simulink model "p_packetizer_test"  (R2012b)
settings: Solver=ode45  StartTime=0.0  StopTime=16384 * 8  RelTol=1e-3
libraries: xbsIndex_r4 x583, casper_library_misc x4
(part 1 of 4)
settings Model: Creator=jackh  LastModifiedBy=jackh

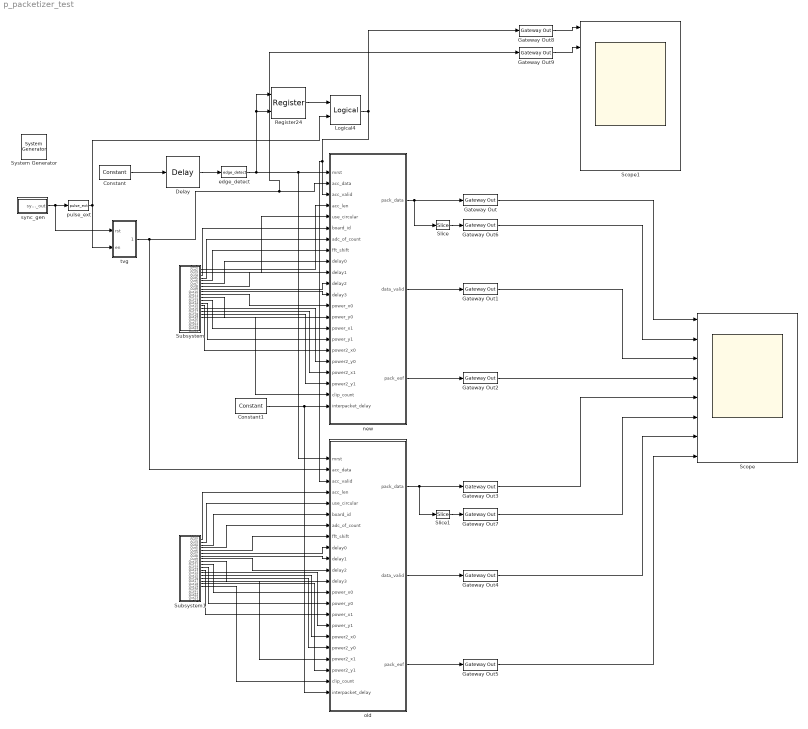
== system p_packetizer_test ==
  " System Generator" : xbsIndex_r4/ System Generator  Tag=genX  xilinxfamily=virtex6  part=xc6vsx475t  speed=-1  package=ff1759  synthesis_tool=XST  clock_wrapper=Clock Enables  directory=./eovsa_corr/sysgen  proj_type=Project Navigator  Synth_file=XST Defaults  Impl_file=ISE Defaults  testbench=off  simulink_period=1  sysclk_period=5  dcm_input_clock_period=100  incr_netlist=off  trim_vbits=Everywhere in SubSystem  dbl_ovrd=According to Block Masks  core_generation=According to Block Masks  run_coregen=off  deprecated_control=off  eval_field=0  block_type=sysgen
      settings: block_version=11.4
  Constant : xbsIndex_r4/Constant  const=1  gui_display_data_type=Boolean  arith_type=Boolean  n_bits=16  bin_pt=14  preci_type=Single  exp_width=8  frac_width=24  explicit_period=on  period=1  equ=P=C  opselect=C  inp2=PCIN>>17  opr=+  inp1=P  carry=CIN  dbl_ovrd=off  block_type=constant
  Constant1 : xbsIndex_r4/Constant  const=5  gui_display_data_type=Fixed-point  arith_type=Unsigned  n_bits=16  bin_pt=0  preci_type=Single  exp_width=8  frac_width=24  explicit_period=on  period=1  equ=P=C  opselect=C  inp2=PCIN>>17  opr=+  inp1=P  carry=CIN  dbl_ovrd=off  block_type=constant
  Delay : xbsIndex_r4/Delay  rst=off  infoeditControl=Selection of Reset will increase slice count due to use of real FFs and instead of SRLs  en=off  latency=3000  dbl_ovrd=off  reg_retiming=off  block_type=delay
  Gateway Out{,1..9} (10 alike) : xbsIndex_r4/Gateway Out  inherit_from_input=off  hdl_port=on  timing_constraint=None  locs_specified=off  LOCs={}  UseAsDAC=off  DACChannel='1'  block_type=gatewayout
  Logical4 : xbsIndex_r4/Logical  logical_function=AND  inputs=2  en=off  latency=0  precision=Full  arith_type=Unsigned  n_bits=16  bin_pt=0  align_bp=on  dbl_ovrd=off  block_type=logical
      settings: block_version=11.4
  Register24 : xbsIndex_r4/Register  init=0  rst=off  en=on  dbl_ovrd=off  block_type=register
  Scope : Scope  NumInputPorts=8
      settings: YMin=0~0~0~0~0~0~0~0  YMax=7e+18~4500~1~1~7e+18~4500~1~1
  Scope1 : Scope  NumInputPorts=8
      settings: YMin=0~0~0~0~0~0~0~0  YMax=7e+18~4500~1~1~7e+18~4500~1~1  SaveName=ScopeData2
  Slice : xbsIndex_r4/Slice  nbits=13  boolean_output=off  mode=Lower Bit Location + Width  bit1=0  base1=MSB of Input  bit0=0  base0=LSB of Input  dbl_ovrd=off  block_type=slice
  Slice1 : xbsIndex_r4/Slice  nbits=13  boolean_output=off  mode=Lower Bit Location + Width  bit1=0  base1=MSB of Input  bit0=0  base0=LSB of Input  dbl_ovrd=off  block_type=slice
  Subsystem : Subsystem
  Subsystem1 : Subsystem
  edge_detect : casper_library_misc/edge_detect  edge=Rising  polarity=Active High  x_in=[0 0.08 0.08 0.16 0.16 0.24 0.24 0.32 0.32 0.4]  y_in="[-1 -1  1  1  1  1  1  1  1  1]"  x_out=[0.6 0.68 0.68 0.76 0.76 0.84 0.84 0.92 0.92 1]  y_out="[-1 -1  1  1 -1 -1 -1 -1 -1 -1]"
  new : Subsystem  mask{header_len=88, n_packets=256, freq_chan=12}
      mask prompts: header_len "Packet header length (bytes)"; n_packets "No. of packets per accumulation"; freq_chan "Total frequency channels ( 2 ^ ? )"
      mask init:
      | data_len = (2 ^ freq_chan) * 4 * (96 / 8 ) / n_packets;
  old : Subsystem  mask{header_len=88, n_packets=256, freq_chan=12}
      mask prompts: header_len "Packet header length (bytes)"; n_packets "No. of packets per accumulation"; freq_chan "Total frequency channels ( 2 ^ ? )"
      mask init:
      | data_len = (2 ^ freq_chan) * 4 * (96 / 8 ) / n_packets;
  pulse_ext : casper_library_misc/pulse_ext  pulse_len=2048
  sync_gen : Subsystem  AncestorBlock=casper_library_misc/sync_gen  mask(sync_gen){sim_acc_len=16, fft_size=2048, fft_simult_inputs=1, pfb_fir_taps=1, reorder_vec=[1], scale=1}
      mask prompts: sim_acc_len "Simulation Accumulation Length"; fft_size "FFT Size"; fft_simult_inputs "Simultaneous Inputs (FFT)"; pfb_fir_taps "Taps in pfb_fir (use 1 if no pfb_fir)"; reorder_vec "Reorder Orders (e.g. [2 2 2])"
      mask help:
      | This block computes the sync period based on system parameters as
      | described in Casper memo.  Detailed descritions of the block's
      | variables can be found in the 'Block Documentation' section of
      | the CASPER wiki.
      mask init:
      | sync_gen_init(gcb, ...
      |     'sim_acc_len', sim_acc_len, ...
      |     'fft_size', fft_size, ...
      |     'fft_simult_inputs', fft_simult_inputs,...
      |     'pfb_fir_taps', pfb_fir_taps, ...
      |     'reorder_vec', reorder_vec, ...
      |     'scale', scale);
      settings: AttributesFormatString=sim_sync_period=32768
      mask Help:
      | SyncPeriod=LCM(reorder_vec)*(acc_num)*(pfb_fir_len)*(fft_size/fft_simult_inputs)
      | 
      | See CASPER sync pulse memo for more details.
  tvg : Subsystem
  wires:
  Constant/1 -> Delay/1
  Delay/1 -> edge_detect/1
  edge_detect/1 -> Register24/2, Register24/1, old/1(mrst), new/1(mrst)
  sync_gen/1(sync_out) -> tvg/1(rst), pulse_ext/1
  pulse_ext/1 -> tvg/2(en), Logical4/2
  Constant1/1 -> old/22(interpacket_delay), new/22(interpacket_delay)
  Subsystem/10(Out10) -> new/12(delay3)
  Subsystem/9(Out9) -> new/11(delay2)
  Subsystem/11(Out11) -> new/13(power_x0)
  Subsystem/8(Out8) -> new/10(delay1)
  Subsystem/12(Out12) -> new/14(power_y0)
  Subsystem/7(Out7) -> new/9(delay0)
  Subsystem/13(Out13) -> new/15(power_x1)
  Subsystem/6(Out6) -> new/8(fft_shift)
  Subsystem/14(Out14) -> new/16(power_y1)
  Subsystem/5(Out5) -> new/7(adc_of_count)
  Subsystem/15(Out15) -> new/17(power2_x0)
  Subsystem/4(Out4) -> new/6(board_id)
  Subsystem/16(Out16) -> new/18(power2_y0)
  Subsystem/3(Out3) -> new/5(use_circular)
  Subsystem/17(Out17) -> new/19(power2_x1)
  Subsystem/2(Out2) -> new/4(acc_len)
  Subsystem/18(Out18) -> new/20(power2_y1)
  Subsystem/19(Out19) -> new/21(clip_count)
  Subsystem1/8(Out8) -> old/10(delay1)
  Subsystem1/7(Out7) -> old/9(delay0)
  Subsystem1/9(Out9) -> old/11(delay2)
  Subsystem1/6(Out6) -> old/8(fft_shift)
  Subsystem1/10(Out10) -> old/12(delay3)
  Subsystem1/5(Out5) -> old/7(adc_of_count)
  Subsystem1/11(Out11) -> old/13(power_x0)
  Subsystem1/4(Out4) -> old/6(board_id)
  Subsystem1/12(Out12) -> old/14(power_y0)
  Subsystem1/3(Out3) -> old/5(use_circular)
  Subsystem1/13(Out13) -> old/15(power_x1)
  Subsystem1/2(Out2) -> old/4(acc_len)
  Subsystem1/14(Out14) -> old/16(power_y1)
  Subsystem1/15(Out15) -> old/17(power2_x0)
  Subsystem1/16(Out16) -> old/18(power2_y0)
  Subsystem1/17(Out17) -> old/19(power2_x1)
  Subsystem1/18(Out18) -> old/20(power2_y1)
  Subsystem1/19(Out19) -> old/21(clip_count)
  new/1(pack_data) -> Slice/1, Gateway Out/1
  new/2(data_valid) -> Gateway Out1/1
  new/3(pack_eof) -> Gateway Out2/1
  old/1(pack_data) -> Slice1/1, Gateway Out3/1
  old/2(data_valid) -> Gateway Out4/1
  old/3(pack_eof) -> Gateway Out5/1
  tvg/1(Out1) -> old/2(acc_data), Gateway Out9/1, new/2(acc_data)
  Slice/1 -> Gateway Out6/1
  Slice1/1 -> Gateway Out7/1
  Gateway Out3/1 -> Scope/5
  Gateway Out7/1 -> Scope/6
  Gateway Out2/1 -> Scope/4
  Gateway Out4/1 -> Scope/7
  Gateway Out1/1 -> Scope/3
  Gateway Out5/1 -> Scope/8
  Gateway Out6/1 -> Scope/2
  Gateway Out/1 -> Scope/1
  Register24/1 -> Logical4/1
  Logical4/1 -> old/3(acc_valid), new/3(acc_valid), Gateway Out8/1
  Gateway Out8/1 -> Scope1/1
  Gateway Out9/1 -> Scope1/2

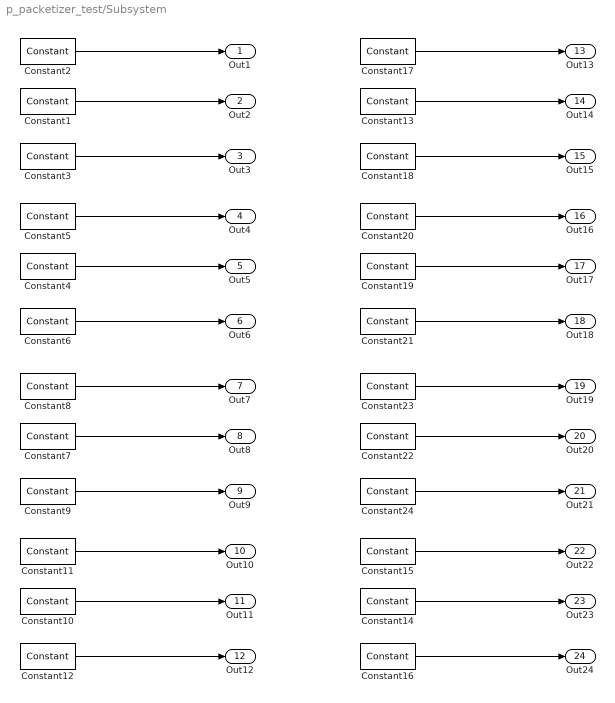
== system p_packetizer_test/Subsystem ==
  Constant{1..24} (24 alike) : xbsIndex_r4/Constant  const=1  gui_display_data_type=Fixed-point  arith_type=Unsigned  n_bits=32  bin_pt=0  preci_type=Single  exp_width=8  frac_width=24  explicit_period=on  period=1  equ=P=C  opselect=C  inp2=PCIN>>17  opr=+  inp1=P  carry=CIN  dbl_ovrd=off  block_type=constant
  Out1 : Outport
  Out2 : Outport  Port=2
  Out3 : Outport  Port=3
  Out4 : Outport  Port=4
  Out5 : Outport  Port=5
  Out6 : Outport  Port=6
  Out7 : Outport  Port=7
  Out8 : Outport  Port=8
  Out9 : Outport  Port=9
  Out10 : Outport  Port=10
  Out11 : Outport  Port=11
  Out12 : Outport  Port=12
  Out13 : Outport  Port=13
  Out14 : Outport  Port=14
  Out15 : Outport  Port=15
  Out16 : Outport  Port=16
  Out17 : Outport  Port=17
  Out18 : Outport  Port=18
  Out19 : Outport  Port=19
  Out20 : Outport  Port=20
  Out21 : Outport  Port=21
  Out22 : Outport  Port=22
  Out23 : Outport  Port=23
  Out24 : Outport  Port=24
  wires:
  Constant2/1 -> Out1/1
  Constant1/1 -> Out2/1
  Constant3/1 -> Out3/1
  Constant5/1 -> Out4/1
  Constant4/1 -> Out5/1
  Constant6/1 -> Out6/1
  Constant8/1 -> Out7/1
  Constant7/1 -> Out8/1
  Constant9/1 -> Out9/1
  Constant11/1 -> Out10/1
  Constant10/1 -> Out11/1
  Constant12/1 -> Out12/1
  Constant17/1 -> Out13/1
  Constant13/1 -> Out14/1
  Constant18/1 -> Out15/1
  Constant20/1 -> Out16/1
  Constant19/1 -> Out17/1
  Constant21/1 -> Out18/1
  Constant23/1 -> Out19/1
  Constant22/1 -> Out20/1
  Constant24/1 -> Out21/1
  Constant15/1 -> Out22/1
  Constant14/1 -> Out23/1
  Constant16/1 -> Out24/1

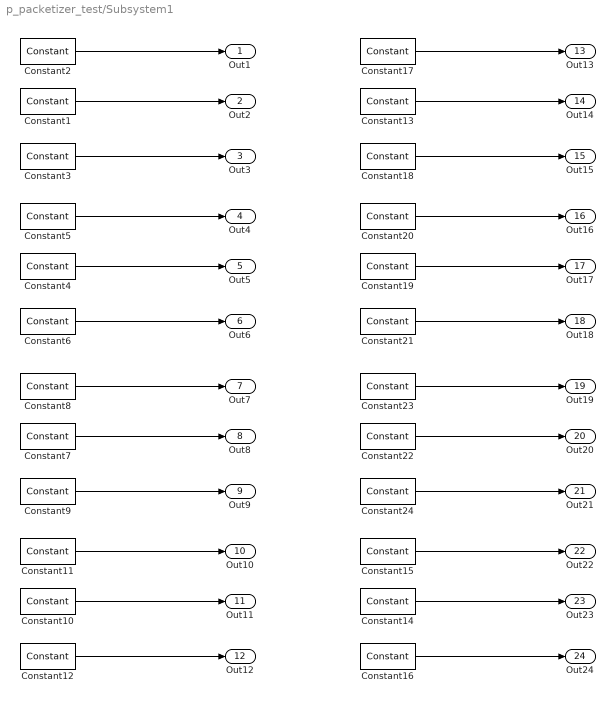
== system p_packetizer_test/Subsystem1 ==
  Constant{1..24} (24 alike) : xbsIndex_r4/Constant  const=1  gui_display_data_type=Fixed-point  arith_type=Unsigned  n_bits=32  bin_pt=0  preci_type=Single  exp_width=8  frac_width=24  explicit_period=on  period=1  equ=P=C  opselect=C  inp2=PCIN>>17  opr=+  inp1=P  carry=CIN  dbl_ovrd=off  block_type=constant
  Out1 : Outport
  Out2 : Outport  Port=2
  Out3 : Outport  Port=3
  Out4 : Outport  Port=4
  Out5 : Outport  Port=5
  Out6 : Outport  Port=6
  Out7 : Outport  Port=7
  Out8 : Outport  Port=8
  Out9 : Outport  Port=9
  Out10 : Outport  Port=10
  Out11 : Outport  Port=11
  Out12 : Outport  Port=12
  Out13 : Outport  Port=13
  Out14 : Outport  Port=14
  Out15 : Outport  Port=15
  Out16 : Outport  Port=16
  Out17 : Outport  Port=17
  Out18 : Outport  Port=18
  Out19 : Outport  Port=19
  Out20 : Outport  Port=20
  Out21 : Outport  Port=21
  Out22 : Outport  Port=22
  Out23 : Outport  Port=23
  Out24 : Outport  Port=24
  wires:
  Constant16/1 -> Out24/1
  Constant14/1 -> Out23/1
  Constant15/1 -> Out22/1
  Constant24/1 -> Out21/1
  Constant22/1 -> Out20/1
  Constant23/1 -> Out19/1
  Constant21/1 -> Out18/1
  Constant19/1 -> Out17/1
  Constant20/1 -> Out16/1
  Constant18/1 -> Out15/1
  Constant13/1 -> Out14/1
  Constant17/1 -> Out13/1
  Constant12/1 -> Out12/1
  Constant10/1 -> Out11/1
  Constant11/1 -> Out10/1
  Constant9/1 -> Out9/1
  Constant7/1 -> Out8/1
  Constant8/1 -> Out7/1
  Constant6/1 -> Out6/1
  Constant4/1 -> Out5/1
  Constant5/1 -> Out4/1
  Constant3/1 -> Out3/1
  Constant1/1 -> Out2/1
  Constant2/1 -> Out1/1

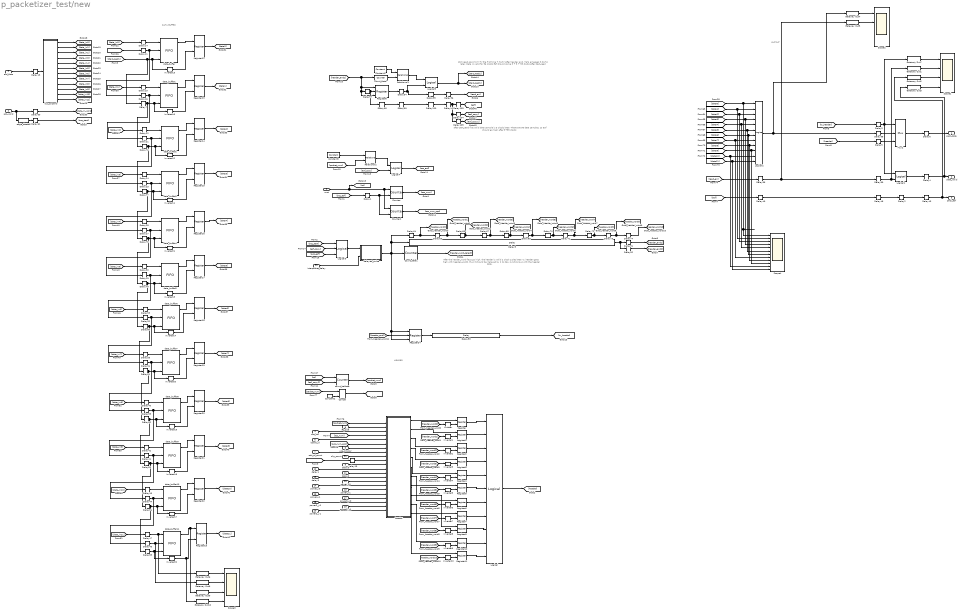
== system p_packetizer_test/new ==
  note: After the header_word flags go high, the header is valid 2 clock cycles later.
      | tx_header goes high with header_word0, thus it should be delayed by 2 to stay synchronous with the header data.
  note: after start_read first valid data sample is 3 clocks later.
      | There are 96 data samples, so eof should go high after 3+95 clocks
  note: start_read goes high for the first time 3 clocks after header_end.
      | Data emerges 3 clocks later.
      | Data is valid for 96 clocks
      | Eof should come 3 + 3 + 95 clocks after start_read
  note: OUTPUT
  note: HEADER
  note: DATA BUFFER
  mrst : Inport
  acc_data : Inport  Port=2
  acc_valid : Inport  Port=3
  acc_len : Inport  Port=4
  use_circular : Inport  Port=5
  board_id : Inport  Port=6
  adc_of_count : Inport  Port=7
  fft_shift : Inport  Port=8
  delay0 : Inport  Port=9
  delay1 : Inport  Port=10
  delay2 : Inport  Port=11
  delay3 : Inport  Port=12
  power_x0 : Inport  Port=13
  power_y0 : Inport  Port=14
  power_x1 : Inport  Port=15
  power_y1 : Inport  Port=16
  power2_x0 : Inport  Port=17
  power2_y0 : Inport  Port=18
  power2_x1 : Inport  Port=19
  power2_y1 : Inport  Port=20
  clip_count : Inport  Port=21
  interpacket_delay : Inport  Port=22
  Concat : xbsIndex_r4/Concat  num_inputs=2  dbl_ovrd=off  block_type=concat
  Constant1 : xbsIndex_r4/Constant  const=0  gui_display_data_type=Fixed-point  arith_type=Unsigned  n_bits=4  bin_pt=0  preci_type=Single  exp_width=8  frac_width=24  explicit_period=on  period=1  equ=P=C  opselect=C  inp2=PCIN>>17  opr=+  inp1=P  carry=CIN  dbl_ovrd=off  block_type=constant
      settings: block_version=11.4
  Constant2 : xbsIndex_r4/Constant  const=0  gui_display_data_type=Fixed-point  arith_type=Unsigned  n_bits=log2( (2 ^ freq_chan) / n_packets )  bin_pt=0  preci_type=Single  exp_width=8  frac_width=24  explicit_period=on  period=1  equ=P=C  opselect=C  inp2=PCIN>>17  opr=+  inp1=P  carry=CIN  dbl_ovrd=off  block_type=constant
      settings: block_version=11.4
  Constant3 : xbsIndex_r4/Constant  const=n_packets - 1  gui_display_data_type=Fixed-point  arith_type=Unsigned  n_bits=ceil( log2( n_packets - 1 ) )  bin_pt=0  preci_type=Single  exp_width=8  frac_width=24  explicit_period=on  period=1  equ=P=C  opselect=C  inp2=PCIN>>17  opr=+  inp1=P  carry=CIN  dbl_ovrd=off  block_type=constant
      settings: block_version=11.4
  Count_data1 : xbsIndex_r4/Counter  cnt_type=Count Limited  cnt_to=header_len / 8 - 1  operation=Up  start_count=0  cnt_by_val=1  arith_type=Unsigned  n_bits=ceil( log2( header_len / 8 - 1 ) )  bin_pt=0  load_pin=off  rst=on  en=off  explicit_period=on  period=1  dbl_ovrd=off  use_behavioral_HDL=on  implementation=Fabric  use_rpm=off  block_type=counter
  Count_data7 : xbsIndex_r4/Counter  cnt_type=Count Limited  cnt_to=11  operation=Up  start_count=0  cnt_by_val=1  arith_type=Unsigned  n_bits=4  bin_pt=0  load_pin=off  rst=on  en=off  explicit_period=on  period=1  dbl_ovrd=off  use_behavioral_HDL=on  implementation=Fabric  use_rpm=off  block_type=counter
  Counter : xbsIndex_r4/Counter  cnt_type=Free Running  cnt_to=Inf  operation=Up  start_count=0  cnt_by_val=1  arith_type=Unsigned  n_bits=32  bin_pt=0  load_pin=off  rst=on  en=on  explicit_period=off  period=1  dbl_ovrd=off  use_behavioral_HDL=off  implementation=DSP48  block_type=counter
      settings: block_version=11.4
  Counter1 : xbsIndex_r4/Counter  cnt_type=Count Limited  cnt_to=49  operation=Up  start_count=0  cnt_by_val=1  arith_type=Unsigned  n_bits=8  bin_pt=0  load_pin=off  rst=on  en=on  explicit_period=off  period=1  dbl_ovrd=off  use_behavioral_HDL=off  implementation=Fabric  block_type=counter
      settings: block_version=11.4
  Delay{1..4,6,9,13..14,32,34,41,43..44,48..49,56,58..59,64..74,95,98..100} (33 alike) : xbsIndex_r4/Delay  rst=off  infoeditControl=Selection of Reset will increase slice count due to use of real FFs and instead of SRLs  en=off  latency=1  dbl_ovrd=off  reg_retiming=on  block_type=delay
      settings: block_version=11.4
  Delay{7,11,15..16,21,23,27,29,39,46,60..61,76..85,91..92,94,102..105} (29 alike) : xbsIndex_r4/Delay  rst=off  infoeditControl=Selection of Reset will increase slice count due to use of real FFs and instead of SRLs  en=off  latency=1  dbl_ovrd=off  reg_retiming=off  block_type=delay
      settings: block_version=11.4
  Delay19 : xbsIndex_r4/Delay  rst=off  infoeditControl=Selection of Reset will increase slice count due to use of real FFs and instead of SRLs  en=off  latency=2  dbl_ovrd=off  reg_retiming=on  block_type=delay
      settings: block_version=11.4
  Delay22 : xbsIndex_r4/Delay  rst=off  infoeditControl=Selection of Reset will increase slice count due to use of real FFs and instead of SRLs  en=off  latency=3  dbl_ovrd=off  reg_retiming=on  block_type=delay
      settings: block_version=11.4
  Delay24 : xbsIndex_r4/Delay  rst=off  infoeditControl=Selection of Reset will increase slice count due to use of real FFs and instead of SRLs  en=off  latency=4  dbl_ovrd=off  reg_retiming=on  block_type=delay
      settings: block_version=11.4
  Delay28 : xbsIndex_r4/Delay  rst=off  infoeditControl=Selection of Reset will increase slice count due to use of real FFs and instead of SRLs  en=off  latency=5  dbl_ovrd=off  reg_retiming=on  block_type=delay
      settings: block_version=11.4
  Delay30 : xbsIndex_r4/Delay  rst=off  infoeditControl=Selection of Reset will increase slice count due to use of real FFs and instead of SRLs  en=off  latency=6  dbl_ovrd=off  reg_retiming=on  block_type=delay
      settings: block_version=11.4
  Delay33 : xbsIndex_r4/Delay  rst=off  infoeditControl=Selection of Reset will increase slice count due to use of real FFs and instead of SRLs  en=off  latency=7  dbl_ovrd=off  reg_retiming=on  block_type=delay
      settings: block_version=11.4
  Delay35 : xbsIndex_r4/Delay  rst=off  infoeditControl=Selection of Reset will increase slice count due to use of real FFs and instead of SRLs  en=off  latency=8  dbl_ovrd=off  reg_retiming=on  block_type=delay
      settings: block_version=11.4
  Delay40 : xbsIndex_r4/Delay  rst=off  infoeditControl=Selection of Reset will increase slice count due to use of real FFs and instead of SRLs  en=off  latency=9  dbl_ovrd=off  reg_retiming=on  block_type=delay
      settings: block_version=11.4
  Delay42 : xbsIndex_r4/Delay  rst=off  infoeditControl=Selection of Reset will increase slice count due to use of real FFs and instead of SRLs  en=off  latency=10  dbl_ovrd=off  reg_retiming=on  block_type=delay
      settings: block_version=11.4
  Delay45 : xbsIndex_r4/Delay  rst=off  infoeditControl=Selection of Reset will increase slice count due to use of real FFs and instead of SRLs  en=off  latency=11  dbl_ovrd=off  reg_retiming=on  block_type=delay
      settings: block_version=11.4
  Delay47 : xbsIndex_r4/Delay  rst=off  infoeditControl=Selection of Reset will increase slice count due to use of real FFs and instead of SRLs  en=off  latency=12  dbl_ovrd=off  reg_retiming=on  block_type=delay
      settings: block_version=11.4
  Delay5 : xbsIndex_r4/Delay  rst=off  infoeditControl=Selection of Reset will increase slice count due to use of real FFs and instead of SRLs  en=off  latency=10  dbl_ovrd=off  reg_retiming=on  block_type=delay
      settings: block_version=11.4
  Delay53 : xbsIndex_r4/Delay  rst=off  infoeditControl=Selection of Reset will increase slice count due to use of real FFs and instead of SRLs  en=off  latency=2  dbl_ovrd=off  reg_retiming=on  block_type=delay
      settings: block_version=11.4
  Delay96 : xbsIndex_r4/Delay  rst=off  infoeditControl=Selection of Reset will increase slice count due to use of real FFs and instead of SRLs  en=off  latency=3  dbl_ovrd=off  reg_retiming=on  block_type=delay
      settings: block_version=11.4
  Delay97 : xbsIndex_r4/Delay  rst=off  infoeditControl=Selection of Reset will increase slice count due to use of real FFs and instead of SRLs  en=off  latency=data_len / 8  dbl_ovrd=off  reg_retiming=off  block_type=delay
      settings: block_version=11.4
  Gateway Out{1..10} (10 alike) : xbsIndex_r4/Gateway Out  inherit_from_input=off  hdl_port=off  timing_constraint=None  locs_specified=off  LOCs={}  UseAsDAC=off  DACChannel='1'  block_type=gatewayout
      settings: infoedit="Gateway out block.  Converts Xilinx fixed point inputs into ouputs of type Simulink integer, double, or fixed point.<br><br>Hardware notes:  In hardware these blocks become top level output ports or are discarded, depending on how they are configured."  block_version=11.4
  Inverter{,1..10} (11 alike) : xbsIndex_r4/Inverter  en=off  latency=0  dbl_ovrd=off  block_type=inv
  Inverter{11..22} (12 alike) : xbsIndex_r4/Inverter  en=off  latency=2  dbl_ovrd=off  block_type=inv
  Logical : xbsIndex_r4/Logical  logical_function=OR  inputs=11  en=off  latency=1  precision=Full  arith_type=Unsigned  n_bits=16  bin_pt=0  align_bp=on  dbl_ovrd=off  block_type=logical
  Logical1 : xbsIndex_r4/Logical  logical_function=OR  inputs=2  en=off  latency=1  precision=Full  arith_type=Unsigned  n_bits=16  bin_pt=0  align_bp=on  dbl_ovrd=off  block_type=logical
      settings: block_version=11.4
  Logical2 : xbsIndex_r4/Logical  logical_function=OR  inputs=12  en=off  latency=1  precision=Full  arith_type=Unsigned  n_bits=16  bin_pt=0  align_bp=on  dbl_ovrd=off  block_type=logical
  Logical4 : xbsIndex_r4/Logical  logical_function=AND  inputs=2  en=off  latency=0  precision=Full  arith_type=Unsigned  n_bits=16  bin_pt=0  align_bp=on  dbl_ovrd=off  block_type=logical
      settings: block_version=11.4
  Logical5 : xbsIndex_r4/Logical  logical_function=AND  inputs=2  en=off  latency=1  precision=Full  arith_type=Unsigned  n_bits=16  bin_pt=0  align_bp=on  dbl_ovrd=off  block_type=logical
      settings: block_version=11.4
  Logical9 : xbsIndex_r4/Logical  logical_function=XOR  inputs=3  en=off  latency=0  precision=Full  arith_type=Unsigned  n_bits=16  bin_pt=0  align_bp=on  dbl_ovrd=off  block_type=logical
      settings: block_version=11.4
  Mux2 : xbsIndex_r4/Mux  inputs=2  en=off  latency=1  precision=Full  arith_type=Unsigned  n_bits=16  bin_pt=14  quantization=Truncate  overflow=Wrap  dbl_ovrd=off  block_type=mux
      settings: block_version=11.4
  Register{,1..7,9..23} (23 alike) : xbsIndex_r4/Register  init=0  rst=on  en=off  dbl_ovrd=off  block_type=register
  Register24 : xbsIndex_r4/Register  init=0  rst=on  en=on  dbl_ovrd=off  block_type=register
  Register8 : xbsIndex_r4/Register  init=0  rst=on  en=on  dbl_ovrd=off  block_type=register
  Relational1 : xbsIndex_r4/Relational  mode=a=b  en=off  latency=1  dbl_ovrd=off  block_type=relational
  Relational2 : xbsIndex_r4/Relational  mode=a=b  en=off  latency=1  dbl_ovrd=off  block_type=relational
  Scope1 : Scope  NumInputPorts=4
      settings: TimeRange=1000  YMin=0~-5~-5~-5  YMax=30~5~5~5
  Scope2 : Scope  NumInputPorts=4
      settings: TimeRange=1000  YMin=0~-5~-5~-5  YMax=1200~5~5~5  SaveName=ScopeData3
  Scope3 : Scope  NumInputPorts=4
      settings: TimeRange=1000  YMin=0~-5~-5~-5  YMax=30~5~5~5  SaveName=ScopeData4
  Scope4 : Scope  NumInputPorts=12
      settings: TimeRange=1000  YMin=0~-5~-5~-5~-5~-5~-5~-5~-5~-5~-5~-5  YMax=1200~5~5~5~5~5~5~5~5~5~5~5  SaveName=ScopeData5
  bus_expand : Subsystem  AncestorBlock=casper_library_flow_control/bus_expand  mask(bus_expand){mode=divisions of equal size, outputNum=12, outputWidth=64, outputBinaryPt=0, outputArithmeticType=0, show_format=off, outputToWorkspace=off, variablePrefix=out, outputToModelAsWell=on}
      mask prompts: outputNum "Number of outputs:"; outputWidth "Output width:"; outputBinaryPt "Output binary point position:"; outputArithmeticType "Output arithmetic type (ufix=0, fix=1, bool=2):"; show_format "Print format string?"; outputToWorkspace "Output to workspace?"; variablePrefix "Variable name prefix:"; outputToModelAsWell "Output to model as well?"
      mask help:
      | Expands a 'bus' made using a bus_create or Xilinx
      | concat block.
      | The input will be divided into the specified number
      | of outputs with the specified arithmetic types.
      | Divisions are made from most significant bit.
      mask init:
      | bus_expand_init(gcb,...
      |     'mode', mode, ...
      |     'outputNum', outputNum, ...
      |     'outputWidth', outputWidth, ...
      |     'outputBinaryPt', outputBinaryPt, ...
      |     'outputArithmeticType', outputArithmeticType, ...
      |     'show_format', show_format, ...
      |     'outputToWorkspace', outputToWorkspace, ...
      |     'variablePrefix', variablePrefix, ...
      |     'outputToModelAsWell', outputToModelAsWell);
      settings: AttributesFormatString=12 outputs
      mask TypeOptions mode: divisions of equal size | divisions of arbitrary size
      mask Callback mode: bus_expand_callback();
      mask Callback outputWidth: bus_expand_callback();
      mask Callback outputToWorkspace: bus_expand_callback();
  count_packets : xbsIndex_r4/Counter  cnt_type=Count Limited  cnt_to=n_packets - 1  operation=Up  start_count=0  cnt_by_val=1  arith_type=Unsigned  n_bits=ceil( log2( n_packets ) )  bin_pt=0  load_pin=off  rst=on  en=on  explicit_period=off  period=1  dbl_ovrd=off  use_behavioral_HDL=off  implementation=DSP48  use_rpm=off  block_type=counter
  data_buffer{,1..11} (12 alike) : xbsIndex_r4/FIFO  mem_type=Block RAM  performance_options=Standard_FIFO  infoedit1=Available only for V4, V5, V6, V7, K7, A7 and Zynq devices.  embedded_registers=on  depth=2K  percent_nbits=1  rst=off  en=off  use_dcount=off  use_percent_full_port=off  use_almost_empty=off  almost_empty_thresh=2  use_almost_full=off  almost_full_thresh=14  dbl_ovrd=off  explicit_period=off  block_type=fifo
      settings: block_version=10.1.3
  delayed_pulse : Subsystem
  edge_detect2 : Subsystem  AncestorBlock=casper_library_misc/edge_detect  mask(edge_detect){edge=Rising, polarity=Active High, x_in=[0 0.08 0.08 0.16 0.16 0.24 0.24 0.32 0.32 0.4], y_in=[-1 -1  1  1  1  1  1  1  1  1], x_out=[0.6 0.68 0.68 0.76 0.76 0.84 0.84 0.92 0.92 1], y_out=[-1 -1  1  1 -1 -1 -1 -1 -1 -1]}
      mask prompts: edge "Edge Type"; polarity "Output Polarity"; x_in "Input X Positions"; y_in "Input Y Positions"; x_out "Output X Positions"; y_out "Output Y Positions"
      mask help: Output is active for one-cycle after each edge of the specified type (i.e. rising, falling or both).
      mask init:
      | edge_detect_init(gcb,...
      |     'edge',edge,...
      |     'polarity',polarity,...
      |     'x_in',x_in,...
      |     'x_out',x_out,...
      |     'y_in',y_in,...
      |     'y_out',y_out);
      | 
      | x_in_num=str2num(getfield(getfield(get_param(gcb,'UserData'),'parameters'),'x_in'));
      | x_out_num=str2num(getfield(getfield(get_param(gcb,'UserData'),'parameters'),'x_out'));
      | y_in_num=str2num(getfield(getfield(get_param(gcb,'UserData'),'parameters'),'y_in'));
      | y_out_num=str2num(getfield(getfield(get_param(gcb,'UserData'),'parameters'),'y_out'));
      settings: AttributesFormatString=|
      | rising edges
      | active high
      mask Help: Output is active for one-cycle after each edge of the specified type (i.e. rising, falling, or both).  Latency is zero.
      mask TypeOptions edge: Rising | Falling | Both
      mask TypeOptions polarity: Active High | Active Low
      mask Display:
      | plot(x_in_num,0.5+y_in_num*0.2);
      | plot(x_out_num,0.5+y_out_num*0.2);
  header : Subsystem
  pack_data : Outport
  data_valid : Outport  Port=2
  pack_eof : Outport  Port=3
  wires:
  Delay14/1 -> data_buffer/1
  Delay11/1 -> Delay16/1, data_buffer/2
  acc_data/1 -> Delay13/1
  Mux2/1 -> Delay6/1
  [eof_copy] -> Logical9/2
  [acc_start] -> Logical9/1
  Count_data1/1 -> [header_word_select]
  Logical1/1 -> Delay4/1
  edge_detect2/1(out) -> Delay61/1
  acc_len/1 -> header/3(acc_len)
  [acc_num] -> header/4(acc_num)
  [acc_num_pps] -> header/6(acc_num_pps)
  use_circular/1 -> header/7(circular)
  Constant3/1 -> Relational2/1
  [packet_num] -> Relational2/2
  Relational2/1 -> Logical4/1
  Logical4/1 -> [acc_eof]
  [acc_eof] -> Logical9/3
  adc_of_count/1 -> header/8(adc_of_count)
  Constant2/1 -> Concat/2
  Concat/1 -> [subband_index]
  [subband_index] -> Delay15/1
  fft_shift/1 -> header/2(fft_shift)
  delay0/1 -> header/11(delay0)
  delay1/1 -> header/12(delay1)
  delay2/1 -> header/13(delay2)
  delay3/1 -> header/14(delay3)
  power_x0/1 -> header/15(power_x0)
  power_y0/1 -> header/16(power_y0)
  power_y1/1 -> header/18(power_y1)
  power_x1/1 -> header/17(power_x1)
  power2_x0/1 -> header/19(power2_x0)
  power2_y0/1 -> header/20(power2_y0)
  power2_x1/1 -> header/21(power2_x1)
  power2_y1/1 -> header/22(power2_y1)
  [data0] -> Scope4/1, Logical2/1
  Delay56/1 -> Gateway Out5/1, Delay59/1
  [eof_copy] -> Logical4/2
  clip_count/1 -> header/9(clip_count)
  Delay3/1 -> Logical1/1, Mux2/1, Gateway Out7/1
  Logical/1 -> [header]
  Delay4/1 -> data_valid/1, Gateway Out3/1
  Delay6/1 -> pack_data/1
  interpacket_delay/1 -> delayed_pulse/2(In2)
  delayed_pulse/1(delayed_eof) -> Register24/1, Register24/3, Delay5/1, Delay64/1, Count_data1/1
  Logical9/1 -> delayed_pulse/1(pack_eof)
  mrst/1 -> Counter/1, Counter1/1, [rst]
  Delay1/1 -> Counter/2, Counter1/2
  Counter1/1 -> [acc_num_pps]
  [acc_eof] -> Delay1/1
  [eof_copy2] -> count_packets/2
  [rst] -> count_packets/1
  [tx_header] -> Delay3/1
  Delay9/1 -> Mux2/3
  bus_expand/1(msb_out12) -> [data_in0]
  bus_expand/2(out11) -> [data_in1]
  bus_expand/3(out10) -> [data_in2]
  bus_expand/4(out9) -> [data_in3]
  bus_expand/5(out8) -> [data_in4]
  bus_expand/6(out7) -> [data_in5]
  bus_expand/7(out6) -> [data_in6]
  bus_expand/8(out5) -> [data_in7]
  bus_expand/9(out4) -> [data_in8]
  bus_expand/10(out3) -> [data_in9]
  bus_expand/11(out2) -> [data_in10]
  bus_expand/12(lsb_out1) -> [data_in11]
  Delay13/1 -> bus_expand/1(bus_in)
  acc_valid/1 -> Delay60/1, edge_detect2/1(in)
  [data_in0] -> Delay14/1
  [data_in_valid] -> Delay11/1
  Delay19/1 -> data_buffer1/1
  Delay16/1 -> Delay21/1, data_buffer1/2
  [data_in1] -> Delay19/1
  Delay22/1 -> data_buffer2/1
  Delay21/1 -> Delay23/1, data_buffer2/2
  [data_in2] -> Delay22/1
  Delay24/1 -> data_buffer3/1
  Delay23/1 -> Delay27/1, data_buffer3/2
  [data_in3] -> Delay24/1
  Delay28/1 -> data_buffer4/1
  Delay27/1 -> Delay29/1, data_buffer4/2
  [data_in4] -> Delay28/1
  Delay30/1 -> data_buffer5/1
  Delay29/1 -> Delay32/1, data_buffer5/2
  [data_in5] -> Delay30/1
  Delay33/1 -> data_buffer6/1
  Delay32/1 -> Delay34/1, data_buffer6/2
  [data_in6] -> Delay33/1
  Delay35/1 -> data_buffer7/1
  Delay34/1 -> Delay39/1, data_buffer7/2
  [data_in7] -> Delay35/1
  Delay40/1 -> data_buffer8/1
  Delay39/1 -> data_buffer8/2, Delay41/1
  [data_in8] -> Delay40/1
  Delay42/1 -> data_buffer9/1
  Delay41/1 -> data_buffer9/2, Delay44/1
  [data_in9] -> Delay42/1
  Delay45/1 -> data_buffer10/1
  Delay44/1 -> data_buffer10/2, Delay46/1
  Delay84/1 -> Delay85/1, Inverter17/1, data_buffer10/3
  [data_in10] -> Delay45/1
  Delay47/1 -> Gateway Out6/1, data_buffer11/1
  Delay46/1 -> Gateway Out8/1, data_buffer11/2
  [data_in11] -> Delay47/1
  [data1] -> Scope4/2, Logical2/2
  [data2] -> Scope4/3, Logical2/3
  [data3] -> Scope4/4, Logical2/4
  [data4] -> Scope4/5, Logical2/5
  [data5] -> Scope4/6, Logical2/6
  [data6] -> Scope4/7, Logical2/7
  [data7] -> Scope4/8, Logical2/8
  [data8] -> Scope4/9, Logical2/9
  [data9] -> Scope4/10, Logical2/10
  [data10] -> Scope4/11, Logical2/11
  [data11] -> Scope4/12, Logical2/12
  count_packets/1 -> [packet_num]
  [packet_num] -> header/1(packet_num)
  [packet_num] -> Concat/1
  Delay2/1 -> Delay43/1
  Logical2/1 -> Gateway Out4/1, Delay58/1
  [read_en] -> Delay56/1
  [header] -> Delay9/1
  Gateway Out7/1 -> Scope1/1
  Gateway Out1/1 -> Scope1/2
  Gateway Out2/1 -> Scope1/3
  Delay58/1 -> Mux2/2
  Delay59/1 -> Logical1/2, Gateway Out1/1
  Gateway Out3/1 -> Scope1/4
  board_id/1 -> header/5(board_id)
  Counter/1 -> [acc_num]
  Delay60/1 -> [data_in_valid]
  Delay61/1 -> [acc_start]
  Delay15/1 -> header/10(subband_index)
  Delay64/1 -> Delay65/1, [header_word0]
  Delay65/1 -> Delay66/1, [header_word1]
  Delay66/1 -> [header_word2], Delay67/1
  Delay67/1 -> [header_word3], Delay68/1
  Delay68/1 -> [header_word4], Delay69/1
  Delay69/1 -> [header_word5], Delay70/1
  Delay70/1 -> [header_word6], Delay71/1
  Delay71/1 -> [header_word7], Delay72/1
  [header_word0] -> Inverter/1
  [header_word1] -> Inverter1/1
  [header_word2] -> Inverter2/1
  [header_word3] -> Inverter3/1
  [header_word4] -> Inverter4/1
  [header_word5] -> Inverter5/1
  [header_word6] -> Inverter6/1
  [header_word7] -> Inverter7/1
  Inverter/1 -> Register/2
  Inverter1/1 -> Register1/2
  Inverter2/1 -> Register2/2
  Inverter3/1 -> Register3/2
  Inverter4/1 -> Register4/2
  Inverter5/1 -> Register5/2
  Inverter6/1 -> Register6/2
  Inverter7/1 -> Register7/2
  header/1(header0) -> Register/1
  header/2(header1) -> Register1/1
  header/3(header2) -> Register2/1
  header/4(header3) -> Register3/1
  header/5(header4) -> Register4/1
  header/6(header5) -> Register5/1
  header/7(header6) -> Register6/1
  header/8(header7) -> Register7/1
  Delay72/1 -> [header_word8], Delay73/1
  Delay73/1 -> [header_word9], Delay74/1
  Register24/1 -> Delay53/1
  Delay74/1 -> [header_word10]
  [header_word8] -> Inverter8/1
  Inverter8/1 -> Register9/2
  [header_word9] -> Inverter9/1
  Inverter9/1 -> Register10/2
  [header_word10] -> Inverter10/1
  Inverter10/1 -> Register11/2
  header/9(header8) -> Register9/1
  header/10(header9) -> Register10/1
  header/11(header10) -> Register11/1
  Register9/1 -> Logical/9
  Register11/1 -> Logical/11
  Register5/1 -> Logical/6
  Register4/1 -> Logical/5
  Register2/1 -> Logical/3
  Register3/1 -> Logical/4
  Register6/1 -> Logical/7
  Register10/1 -> Logical/10
  Register7/1 -> Logical/8
  Register1/1 -> Logical/2
  Register/1 -> Logical/1
  Delay5/1 -> Delay92/1, Delay91/1
  [start_read1] -> Delay7/1, Inverter13/1, data_buffer/3
  Register12/1 -> [data0]
  Inverter13/1 -> Register12/2
  Delay7/1 -> Delay76/1, Inverter16/1, data_buffer1/3
  Delay76/1 -> Delay77/1, Inverter12/1, data_buffer2/3
  Delay77/1 -> Delay78/1, Inverter11/1, data_buffer3/3
  Delay78/1 -> Delay79/1, Inverter21/1, data_buffer4/3
  Delay79/1 -> Delay80/1, Inverter15/1, data_buffer5/3
  Delay80/1 -> Delay81/1, Inverter14/1, data_buffer6/3
  Delay81/1 -> Delay82/1, Inverter20/1, data_buffer7/3
  Delay82/1 -> Delay83/1, Inverter19/1, data_buffer8/3
  Delay83/1 -> Delay84/1, Inverter18/1, data_buffer9/3
  Delay85/1 -> Inverter22/1, data_buffer11/3
  Register13/1 -> [data1]
  Inverter16/1 -> Register13/2
  Register14/1 -> [data2]
  Inverter12/1 -> Register14/2
  Register15/1 -> [data3]
  Inverter11/1 -> Register15/2
  Register16/1 -> [data4]
  Inverter21/1 -> Register16/2
  Register17/1 -> [data5]
  Inverter15/1 -> Register17/2
  Register18/1 -> [data6]
  Inverter14/1 -> Register18/2
  Register19/1 -> [data7]
  Inverter20/1 -> Register19/2
  Register20/1 -> [data8]
  Inverter19/1 -> Register20/2
  Register21/1 -> [data9]
  Inverter18/1 -> Register21/2
  Register22/1 -> [data10]
  Inverter17/1 -> Register22/2
  Register23/1 -> [data11]
  Inverter22/1 -> Gateway Out10/1, Register23/2
  Delay43/1 -> pack_eof/1, Gateway Out2/1
  Delay48/1 -> Delay2/1
  Delay49/1 -> Delay48/1
  [eof] -> Delay49/1
  Delay53/1 -> [tx_header]
  data_buffer6/1 -> Register18/1
  Delay91/1 -> [header_end1]
  Delay92/1 -> [header_end2]
  Count_data7/1 -> Relational1/2
  [header_end1] -> Delay97/1, Register8/3, Register8/1, Count_data7/1
  Constant1/1 -> Relational1/1
  Relational1/1 -> Logical5/1
  Register8/1 -> Delay94/1
  Logical5/1 -> [start_read2], [start_read1]
  Delay94/1 -> Delay95/1, Logical5/2
  Delay95/1 -> Delay96/1
  Delay96/1 -> [read_en]
  Delay97/1 -> Delay98/1, Register8/2
  Delay98/1 -> Delay99/1
  Delay99/1 -> Delay100/1
  Delay100/1 -> Delay102/1
  Delay102/1 -> Delay103/1, Delay104/1, Delay105/1
  Delay103/1 -> [eof]
  Delay104/1 -> [eof_copy]
  Delay105/1 -> [eof_copy2]
  [header_end2] -> Register24/2
  Gateway Out4/1 -> Scope2/1
  Gateway Out5/1 -> Scope2/2
  Gateway Out6/1 -> Scope3/1
  Gateway Out8/1 -> Scope3/2
  Gateway Out9/1 -> Scope3/3
  Gateway Out10/1 -> Scope3/4
  data_buffer/1 -> Register12/1
  data_buffer1/1 -> Register13/1
  data_buffer2/1 -> Register14/1
  data_buffer3/1 -> Register15/1
  data_buffer4/1 -> Register16/1
  data_buffer5/1 -> Register17/1
  data_buffer11/1 -> Gateway Out9/1, Register23/1
  data_buffer7/1 -> Register19/1
  data_buffer8/1 -> Register20/1
  data_buffer9/1 -> Register21/1
  data_buffer10/1 -> Register22/1
